simulink model "msd_resonant_frequency_seeking_DT_vanishing_dither"  (R2024b)
settings: Solver=ode4  StartTime=0.0  StopTime=Tfin  FixedStep=Ts_sim  RelTol=1e-3
values from neighbouring files (symbols this model uses):
  A_cmd = 1    [msd_resonant_frequency_seeking_CT_run.m]    (also in msd_resonant_frequency_seeking_DT_run.m; msd_resonant_frequency_seeking_DT_vanishing_dither_run.m)
  A_esc_d = 1    [msd_resonant_frequency_seeking_CT_run.m]    (also in msd_resonant_frequency_seeking_DT_run.m = 1.2; msd_resonant_frequency_seeking_DT_vanishing_dither_run.m = 1.2)
  A_esc_m_0 = 1.2    [msd_resonant_frequency_seeking_DT_vanishing_dither_run.m]
  alpha_m = 0.1    [msd_resonant_frequency_seeking_DT_vanishing_dither_run.m]
  c = 2    [msd_frequency_response_magnitude.m]    (also in msd_resonant_frequency_seeking_CT_run.m; msd_resonant_frequency_seeking_DT_run.m; msd_resonant_frequency_seeking_DT_vanishing_dither_run.m)
  delta_m = 0.002    [msd_resonant_frequency_seeking_DT_vanishing_dither_run.m]
  k = 1000    [msd_frequency_response_magnitude.m]    (also in msd_resonant_frequency_seeking_CT_run.m; msd_resonant_frequency_seeking_DT_run.m; msd_resonant_frequency_seeking_DT_vanishing_dither_run.m)
  k_en = floor(t_en/Ts_esc)    [msd_resonant_frequency_seeking_DT_vanishing_dither_run.m]
  K_esc = 2.5    [msd_resonant_frequency_seeking_CT_run.m]    (also in msd_resonant_frequency_seeking_DT_run.m = 2; msd_resonant_frequency_seeking_DT_vanishing_dither_run.m)
  K_g = 500    [msd_resonant_frequency_seeking_CT_run.m]    (also in msd_resonant_frequency_seeking_DT_run.m; msd_resonant_frequency_seeking_DT_vanishing_dither_run.m)
  l_rms = 2000    [msd_resonant_frequency_seeking_DT_run.m]    (also in msd_resonant_frequency_seeking_DT_vanishing_dither_run.m = 100)
  lambda_m = 0.025    [msd_resonant_frequency_seeking_DT_vanishing_dither_run.m]
  lambda_osc = 1    [msd_resonant_frequency_seeking_CT_run.m]    (also in msd_resonant_frequency_seeking_DT_run.m; msd_resonant_frequency_seeking_DT_vanishing_dither_run.m)
  m = 1    [msd_frequency_response_magnitude.m]    (also in msd_resonant_frequency_seeking_CT_run.m; msd_resonant_frequency_seeking_DT_run.m; msd_resonant_frequency_seeking_DT_vanishing_dither_run.m)
  omega_cmd_0 = 20    [msd_resonant_frequency_seeking_CT_run.m]    (also in msd_resonant_frequency_seeking_DT_run.m; msd_resonant_frequency_seeking_DT_vanishing_dither_run.m)
  omega_esc = 1    [msd_resonant_frequency_seeking_CT_run.m]    (also in msd_resonant_frequency_seeking_DT_run.m; msd_resonant_frequency_seeking_DT_vanishing_dither_run.m = 4)
  omega_h = 2    [msd_resonant_frequency_seeking_CT_run.m]    (also in msd_resonant_frequency_seeking_DT_run.m = 0.1; msd_resonant_frequency_seeking_DT_vanishing_dither_run.m = 3)
  omega_l = 4    [msd_resonant_frequency_seeking_CT_run.m]    (also in msd_resonant_frequency_seeking_DT_run.m; msd_resonant_frequency_seeking_DT_vanishing_dither_run.m = 10)
  t_en = 2*(l_rms + 1)*Ts    (= 4.002)    [msd_resonant_frequency_seeking_DT_run.m]    (also in msd_resonant_frequency_seeking_DT_vanishing_dither_run.m = 0.202)
  Ts = 0.001    [msd_resonant_frequency_seeking_CT_run.m]    (also in msd_resonant_frequency_seeking_DT_run.m; msd_resonant_frequency_seeking_DT_vanishing_dither_run.m; nonlinear_oscillator_frequency_switch_test.m)
  Ts_esc = 0.1    [msd_resonant_frequency_seeking_DT_run.m]    (also in msd_resonant_frequency_seeking_DT_vanishing_dither_run.m)
  x0 = [0;0]    [msd_resonant_frequency_seeking_CT_run.m]    (also in msd_resonant_frequency_seeking_DT_run.m; msd_resonant_frequency_seeking_DT_vanishing_dither_run.m; nonlinear_oscillator_frequency_switch_test.m = [0.0; 1.0])
  x_osc_0 = [0; A_cmd]    [msd_resonant_frequency_seeking_DT_run.m]    (also in msd_resonant_frequency_seeking_DT_vanishing_dither_run.m)
  x_rms_0 = 0.00    (= 0)    [msd_resonant_frequency_seeking_DT_run.m]    (also in msd_resonant_frequency_seeking_DT_vanishing_dither_run.m)
undefined symbols (not defined in the file or in its folder): dspblkCoreblockFVToolHelper, gcbh
settings Model: Creator=Juan Augusto Paredes  LastModifiedBy=Juan Augusto Paredes
settings RTWCC: GPUComputeCapability=3.5

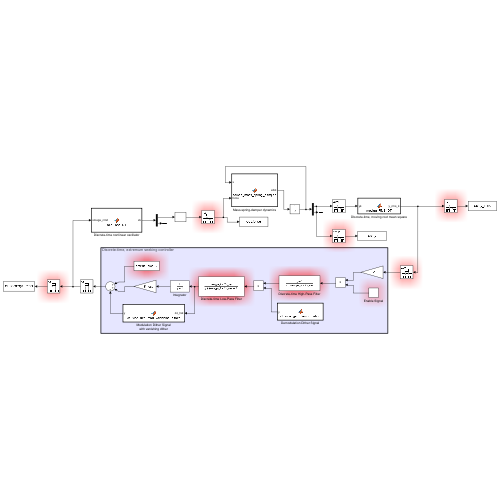
[thumbnail: Simulink's stored preview of the top-level diagram]
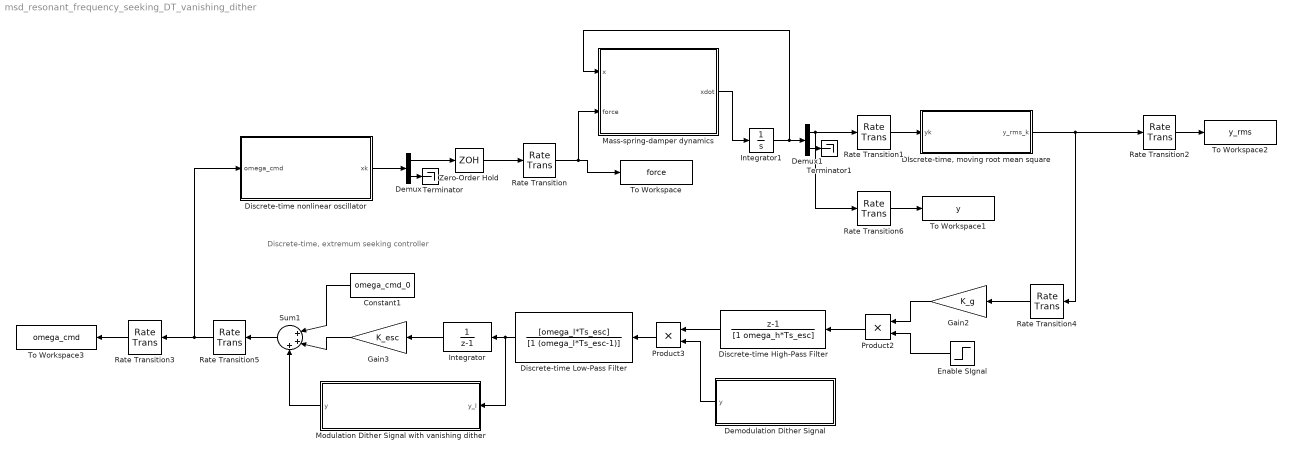
== system msd_resonant_frequency_seeking_DT_vanishing_dither ==
  note: Discrete-time, extremum seeking controller
  Constant1 : Constant  Value=omega_cmd_0  SampleTime=Ts_esc
  "DIscrete-time, moving root mean square" : MATLAB Function  TreatAsAtomicUnit=on
  Demodulation Dither Signal : MATLAB Function  TreatAsAtomicUnit=on
  Demux : Demux  Outputs=2
  Demux1 : Demux  Outputs=2
  Discrete-time High-Pass Filter : DiscreteTransferFcn  LoadFcn=dspblkCoreblockFVToolHelper(gcbh,'load');  Numerator=[1 -1]  Denominator=[1 omega_h*Ts_esc]
      settings: CopyFcn=dspblkCoreblockFVToolHelper(gcbh,'copy');  DeleteFcn=dspblkCoreblockFVToolHelper(gcbh,'close');  ModelCloseFcn=dspblkCoreblockFVToolHelper(gcbh,'close');  PreSaveFcn=dspblkCoreblockFVToolHelper(gcbh,'presave');  PostSaveFcn=dspblkCoreblockFVToolHelper(gcbh,'postsave');  CloseFcn=dspblkCoreblockFVToolHelper(gcbh,'close');
  Discrete-time Low-Pass Filter : DiscreteTransferFcn  LoadFcn=dspblkCoreblockFVToolHelper(gcbh,'load');  Numerator=[omega_l*Ts_esc]  Denominator=[1 (omega_l*Ts_esc-1)]
      settings: CopyFcn=dspblkCoreblockFVToolHelper(gcbh,'copy');  DeleteFcn=dspblkCoreblockFVToolHelper(gcbh,'close');  ModelCloseFcn=dspblkCoreblockFVToolHelper(gcbh,'close');  PreSaveFcn=dspblkCoreblockFVToolHelper(gcbh,'presave');  PostSaveFcn=dspblkCoreblockFVToolHelper(gcbh,'postsave');  CloseFcn=dspblkCoreblockFVToolHelper(gcbh,'close');
  Discrete-time nonlinear oscillator : MATLAB Function  TreatAsAtomicUnit=on
  Enable SIgnal : Step  Time=t_en  SampleTime=Ts_esc
  Gain2 : Gain  Gain=K_g
  Gain3 : Gain  Gain=K_esc
  Integrator : DiscreteTransferFcn  LoadFcn=dspblkCoreblockFVToolHelper(gcbh,'load');  Denominator=[1 -1]
      settings: CopyFcn=dspblkCoreblockFVToolHelper(gcbh,'copy');  DeleteFcn=dspblkCoreblockFVToolHelper(gcbh,'close');  ModelCloseFcn=dspblkCoreblockFVToolHelper(gcbh,'close');  PreSaveFcn=dspblkCoreblockFVToolHelper(gcbh,'presave');  PostSaveFcn=dspblkCoreblockFVToolHelper(gcbh,'postsave');  CloseFcn=dspblkCoreblockFVToolHelper(gcbh,'close');
  Integrator1 : Integrator  InitialCondition=x0
  Mass-spring-damper dynamics : MATLAB Function  TreatAsAtomicUnit=on
  Modulation Dither Signal with vanishing dither : MATLAB Function  TreatAsAtomicUnit=on
  Product2 : Product
  Product3 : Product
  Rate Transition : RateTransition  OutPortSampleTime=Ts_sim
  Rate Transition1 : RateTransition  OutPortSampleTime=Ts
  Rate Transition2 : RateTransition  OutPortSampleTime=Ts_sim
  Rate Transition3 : RateTransition  InitialCondition=omega_cmd_0  OutPortSampleTime=Ts_sim
  Rate Transition4 : RateTransition  OutPortSampleTime=Ts_esc
  Rate Transition5 : RateTransition  InitialCondition=omega_cmd_0  OutPortSampleTime=Ts
  Rate Transition6 : RateTransition  OutPortSampleTime=Ts_sim
  Sum1 : Sum  Inputs=|+++
  Terminator : Terminator
  Terminator1 : Terminator
  To Workspace : ToWorkspace  VariableName=force  SampleTime=-1
  To Workspace1 : ToWorkspace  VariableName=y  SampleTime=-1
  To Workspace2 : ToWorkspace  VariableName=y_rms  SampleTime=-1
  To Workspace3 : ToWorkspace  VariableName=omega_cmd  SampleTime=-1
  Zero-Order Hold : ZeroOrderHold  SampleTime=Ts
  wires:
  Demux/2 -> Terminator/1
  Mass-spring-damper dynamics/1(xdot) -> Integrator1/1
  Integrator1/1 -> Demux1/1, Mass-spring-damper dynamics/1(x)
  Demux1/2 -> Terminator1/1
  Demux1/1 -> Rate Transition6/1, Rate Transition1/1
  Demux/1 -> Zero-Order Hold/1
  Rate Transition/1 -> To Workspace/1, Mass-spring-damper dynamics/2(force)
  Zero-Order Hold/1 -> Rate Transition/1
  Discrete-time nonlinear oscillator/1(xk) -> Demux/1
  Rate Transition1/1 -> "DIscrete-time, moving root mean square"/1(yk)
  Rate Transition2/1 -> To Workspace2/1
  "DIscrete-time, moving root mean square"/1(y_rms_k) -> Rate Transition4/1, Rate Transition2/1
  Rate Transition3/1 -> To Workspace3/1
  Rate Transition5/1 -> Rate Transition3/1, Discrete-time nonlinear oscillator/1(omega_cmd)
  Rate Transition6/1 -> To Workspace1/1
  Sum1/1 -> Rate Transition5/1
  Rate Transition4/1 -> Gain2/1
  Constant1/1 -> Sum1/1
  Gain3/1 -> Sum1/2
  Gain2/1 -> Product2/1
  Modulation Dither Signal with vanishing dither/1(y) -> Sum1/3
  Product3/1 -> Discrete-time Low-Pass Filter/1
  Discrete-time Low-Pass Filter/1 -> Modulation Dither Signal with vanishing dither/1(y_l), Integrator/1
  Product2/1 -> Discrete-time High-Pass Filter/1
  Integrator/1 -> Gain3/1
  Demodulation Dither Signal/1(y) -> Product3/2
  Enable SIgnal/1 -> Product2/2
  Discrete-time High-Pass Filter/1 -> Product3/1

== matlab function msd_resonant_frequency_seeking_DT_vanishing_dither/Mass-spring-damper dynamics ==
  settings: updateMethod=CONTINUOUS
  data: x input size=2; xdot output size=2; force input size=1; m parameter size=1; k parameter size=1; c parameter size=1
function xdot = forced_mass_spring_damper(x,force, m, k, c)
    xdot = [0 1; -k/m -c/m]*x + [0;1/m]*force;
end

== matlab function msd_resonant_frequency_seeking_DT_vanishing_dither/Modulation Dither Signal with vanishing dither ==
  settings: updateMethod=DISCRETE  sampleTime=Ts_esc
  data: y_l input size=1; y output size=1; A_esc_m_0 parameter size=1; omega_esc parameter size=1; Ts_esc parameter size=1; delta_m parameter size=1; alpha_m parameter size=1; lambda_m parameter size=1; k_en parameter size=1
function y = dt_sine_gen_mod_vanishing_dither(y_l, A_esc_m_0, omega_esc, Ts_esc, delta_m, alpha_m, lambda_m, k_en)
    
    persistent kk A_esc_m_k
    if isempty(kk)
        kk = 0;
        A_esc_m_k = A_esc_m_0;
    end
    
    if (kk >= k_en)
       A_esc_m_k = A_esc_m_k + double(norm(y_l) > delta_m)*(-alpha_m*y_l) + double(norm(y_l) <= delta_m)*(-lambda_m*A_esc_m_k);
    end

    y = A_esc_m_k*sin(omega_esc*Ts_esc*kk);
    kk = kk + 1;
    
end

== matlab function msd_resonant_frequency_seeking_DT_vanishing_dither/Demodulation Dither Signal ==
  settings: updateMethod=DISCRETE  sampleTime=Ts_esc
  data: y output size=1; omega_esc parameter size=1; Ts_esc parameter size=1; A_esc_d parameter size=1
function y = dt_sine_gen_demodulation(omega_esc, Ts_esc, A_esc_d)
    
    persistent kk
    if isempty(kk)
        kk = 0;
    end
    y = A_esc_d*sin(omega_esc*Ts_esc*kk);
    kk = kk + 1;
    
end

== matlab function msd_resonant_frequency_seeking_DT_vanishing_dither/Discrete-time nonlinear oscillator ==
  settings: updateMethod=DISCRETE  sampleTime=Ts
  data: omega_cmd input size=1; xk output size=2; lambda_osc parameter size=1; A_cmd parameter size=1; Ts parameter size=1; x_osc_0 parameter size=2
function xk = nonl_osc_DT(omega_cmd, lambda_osc, A_cmd, Ts, x_osc_0)
    % Discrete-time, nonlinear oscillator update equations

    persistent xkm1
    if isempty(xkm1)
        xkm1 = x_osc_0;
    end
    
    aa = cos(omega_cmd*Ts);
    bb = sin(omega_cmd*Ts);
    Omega = [aa bb; -bb aa];
    xk = (Omega - lambda_osc*(xkm1.'*xkm1 - A_cmd^2)*eye(2))*xkm1;
    xkm1 = xk;

end

== matlab function msd_resonant_frequency_seeking_DT_vanishing_dither/DIscrete-time, moving root mean square ==
  settings: updateMethod=DISCRETE  sampleTime=Ts
  data: yk input size=1; y_rms_k output size=1; l_rms parameter size=1; x_rms_0 parameter size=1
function y_rms_k = moving_RMS_DT(yk, l_rms, x_rms_0)

    % Discrete-time, moving root mean square update equations
    persistent x_rms_km1
    if isempty(x_rms_km1)
        x_rms_km1 = x_rms_0;
    end
    x_rms_k = x_rms_km1 + (yk.^2-x_rms_km1)/(l_rms + 1);
    y_rms_k = sqrt(x_rms_k);
    x_rms_km1 = x_rms_k;

end
